simulink model "Suspension_tractor_V2"  (R2017b)
settings: Solver=VariableStepAuto  StartTime=0.0  StopTime=92  RelTol=1e-3
undefined symbols (not defined in the file): dc, ks, kt, m, mu
libraries: simulink x1
settings Model: Creator=mm395  LastModifiedBy=mm395

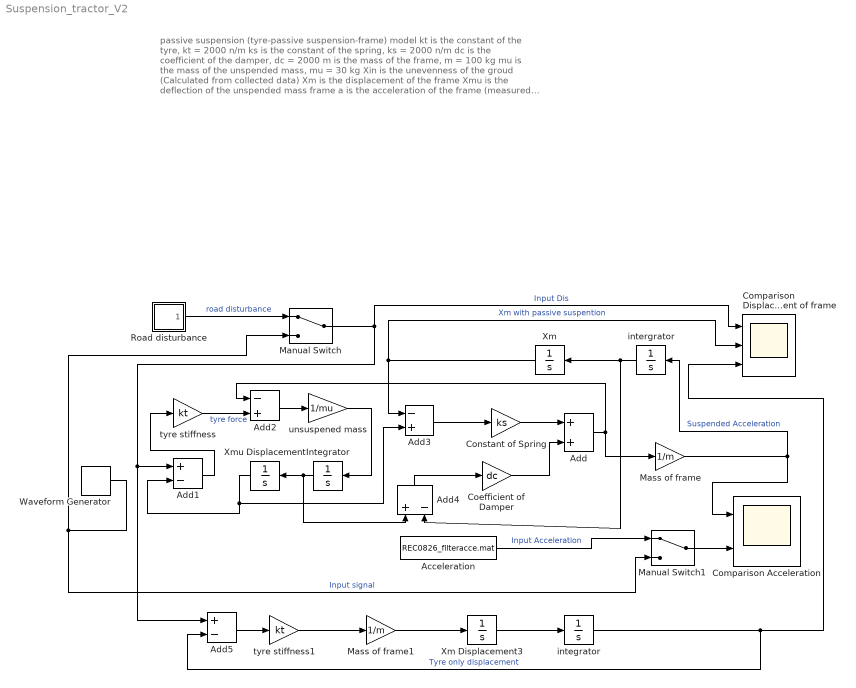
== system Suspension_tractor_V2 ==
  note: passive suspension (tyre-passive suspension-frame) model
      | kt is the constant of the tyre, kt = 2000 n/m
      | ks is the constant of the spring, ks = 2000 n/m
      | dc is the coefficient of the damper, dc = 2000
      | m is the mass of the frame, m = 100 kg
      | mu is the mass of the unspended mass, mu = 30 kg
      | Xin is the unevenness of the groud (Calculated from collected data)
      | Xm is the displacement of the frame
      | Xmu is the deflection of the unspended mass frame
      | a is the acceleration of the frame (measured by accelerometer)
      | a1 is the acceleration of the unsprund mass
      |
      | mu*a1 = (Xin - Xmu)*kt - (Xmu - Xm)*ks - d(Xmu - Xm)/dt * dc
      | m*a = (Xmu - Xm)*ks + d(Xmu - Xm)/dt * dc
      |
      | Designed by: Mengbin Min 24/01/2018
      | Checked by: Shen Hin Lim 24/01/2018
  Acceleration : FromFile  FileName=REC0826_filteracce.mat  SampleTime=1/3200  ExtrapolationBeforeFirstDataPoint=Hold first value  ExtrapolationAfterLastDataPoint=Hold last value
  Add : Sum
  Add1 : Sum  Inputs=+-
  Add2 : Sum  Inputs=-+
  Add3 : Sum  Inputs=-+
  Add4 : Sum  Inputs=+-
  Add5 : Sum  Inputs=+-
  Coefficient of Damper : Gain  Gain=dc
  Comparison Acceleration : Scope  NumInputPorts=2
  Comparison Displacement of frame : Scope  NumInputPorts=3
  Constant of Spring : Gain  Gain=ks
  Integrator : Integrator
  Manual Switch : ManualSwitch
  Manual Switch1 : ManualSwitch
  Mass of frame : Gain  Gain=1/m
  Mass of frame1 : Gain  Gain=1/m
  Road disturbance : Subsystem
  Waveform Generator : simulink/Sources/Waveform Generator  OutMin=[]  OutMax=[]  OutDataTypeStr=double  SelectedSignal=2  Signals=step(1,0,1)#sin(1,1,0)#square(1,1,0,10)  BlockNames=MultiportSwitch_d8e04bd528e6447#MultiportSwitch_56c6f1ec4f694dc#MultiportSwitch_6fb3fe029376448  SampleTime=0.1
      settings: SourceProductName=Simulink
  Xm : Integrator
  Xm Displacement3 : Integrator
  Xmu Displacement : Integrator
  integrator : Integrator
  intergrator : Integrator
  tyre stiffness : Gain  Gain=kt
  tyre stiffness1 : Gain  Gain=kt
  unsuspened mass : Gain  Gain=1/mu
  wires:
  Xmu Displacement/1 -> Add1/2, Add3/2
  Add1/1 -> tyre stiffness/1
  Constant of Spring/1 -> Add/1
  Road disturbance/1(Out1) -> Manual Switch/1  "road disturbance"
  Mass of frame/1 -> intergrator/1, Comparison Acceleration/1  "Suspended Acceleration"
  Add/1 -> Add2/1, Mass of frame/1
  Coefficient of Damper/1 -> Add/2
  tyre stiffness/1 -> Add2/2  "tyre force"
  Add2/1 -> unsuspened mass/1
  unsuspened mass/1 -> Integrator/1
  Integrator/1 -> Xmu Displacement/1, Add4/1
  Add3/1 -> Constant of Spring/1
  intergrator/1 -> Add4/2, Xm/1
  Add4/1 -> Coefficient of Damper/1
  Xm/1 -> Add3/1, Comparison Displacement of frame/2  "Xm with passive suspention"
  Add5/1 -> tyre stiffness1/1
  tyre stiffness1/1 -> Mass of frame1/1
  Mass of frame1/1 -> Xm Displacement3/1
  Xm Displacement3/1 -> integrator/1
  integrator/1 -> Add5/2, Comparison Displacement of frame/3  "Tyre only displacement"
  Manual Switch/1 -> Add5/1, Add1/1, Comparison Displacement of frame/1  "Input Dis"
  Acceleration/1 -> Manual Switch1/1  "Input Acceleration"
  Manual Switch1/1 -> Comparison Acceleration/2
  Waveform Generator/1 -> Manual Switch/2, Manual Switch1/2  "Input signal"

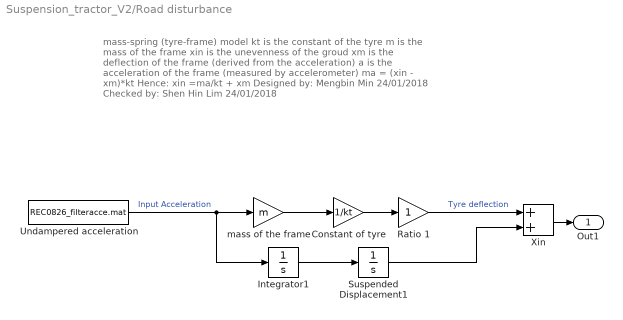
== system Suspension_tractor_V2/Road disturbance ==
  note: mass-spring (tyre-frame) model
      | kt is the constant of the tyre
      | m is the mass of the frame
      | xin is the unevenness of the groud
      | xm is the deflection of the frame (derived from the acceleration)
      | a is the acceleration of the frame (measured by accelerometer)
      |
      | ma = (xin - xm)*kt
      | Hence: xin =ma/kt + xm
      |
      | Designed by: Mengbin Min 24/01/2018
      | Checked by: Shen Hin Lim 24/01/2018
  Constant of tyre : Gain  Gain=1/kt
  Integrator1 : Integrator
  Ratio 1 : Gain
  Suspended Displacement1 : Integrator
  Undampered acceleration : FromFile  FileName=REC0826_filteracce.mat  SampleTime=1/3200  ExtrapolationBeforeFirstDataPoint=Hold first value  ExtrapolationAfterLastDataPoint=Hold last value
  Xin : Sum
  mass of the frame : Gain  Gain=m
  Out1 : Outport
  wires:
  Xin/1 -> Out1/1
  Suspended Displacement1/1 -> Xin/2
  Constant of tyre/1 -> Ratio 1/1
  Ratio 1/1 -> Xin/1  "Tyre deflection"
  mass of the frame/1 -> Constant of tyre/1
  Integrator1/1 -> Suspended Displacement1/1
  Undampered acceleration/1 -> Integrator1/1, mass of the frame/1  "Input Acceleration"
